simulink model "sm_vehicle_2axle_heave_roll_vtk"  (R2023b)
settings: Solver=ode1  StartTime=0.0  StopTime=inf  FixedStep=0.001  MaxStep=0.2  RelTol=1e-3  AbsTol=1e-3  EnableMultiTasking=on
PostLoadFcn:
  | if any(exist('dsrtsu_mdlpostloadfcn', 'file') ~= 0), dsrtsu_mdlpostloadfcn('Execute', bdroot); end
  | sm_vehicle_2axle_heave_roll_param
  | sm_vehicle_2axle_heave_roll_scene
  | sm_vehicle_2axle_heave_roll_config_maneuver(bdroot,VehicleData,'external');
InitFcn:
  | , if any(exist('rtifpga_mdlclblib', 'file') ~= 0), rtifpga_mdlclblib('Init', bdroot); end,
  | , if any(exist('dsmpb_private', 'file') ~= 0), dsmpb_private('dsmpb_mdlclblib', 'Init', bdroot); end,
StartFcn:
  | tic
StopFcn:
  | Elapsed_Sim_Time = toc;
undefined symbols (not defined in the file): InitVehicle, Maneuver, SceneData, trqFL, trqFR, trqRL, trqRR, VehicleData, VehicleData_P, X, Y, Z
libraries: sm_lib x62, nesl_utility x35, sm_vehicle_utilities_lib x18
(part 1 of 3)
PreSaveFcn:
  | , if any(exist('dsmpb_private', 'file') ~= 0), dsmpb_private('dsmpb_mdlclblib', 'PreSave', bdroot); end,
CloseFcn:
  | , if any(exist('dsmpb_private', 'file') ~= 0), dsmpb_private('dsmpb_mdlclblib', 'Close', bdroot); end,
  | try,close(h1_sm_vehicle_2axle_heave_roll),end
  | clear h1_sm_vehicle_2axle_heave_roll
  | try,close(h2_sm_vehicle_2axle_heave_roll),end
  | clear h2_sm_vehicle_2axle_heave_roll
  | try,close(h3_sm_vehicle_2axle_heave_roll),end
  | clear h3_sm_vehicle_2axle_heave_roll
  | 
  | 
  | clear simlog_sm_vehicle_2axle_heave_roll
  | clear logsout_sm_vehicle_2axle_heave_roll
Description:
  | Vehicle Dynamics, 14 DOF Model (Heave and Roll DOFs Per Axle)
  | 
  | Copyright 2022-2023 The MathWorks, Inc.
settings Model: DSMPB_ID_DATA={}  DSRTSU_INTERNAL_RTIFPGA=210  DSRTSU_INTERNAL_RTISTBM_VER=23.2  TunableVars=InitVehicle  TunableVarsStorageClass=ExportedGlobal  Creator=smiller  LastModifiedBy=matlabuser2
settings SolverCC: AutoScaleAbsTol=off  AlgebraicLoopSolver=TrustRegion
settings DataIOCC: SaveFormat=Array  SaveOutput=off  ReturnWorkspaceOutputs=off  SignalLoggingName=logsout_sm_vehicle_2axle_heave_roll_vtk  OutputTimes=[0:0.01:10]
settings OptimizationCC: DefaultParameterBehavior=Inlined  EnhancedBackFolding=on  ExpressionDepthLimit=2147483647  OptimizeBlockOrder=speed  DifferentSizesBufferReuse=on  OptimizationCustomize=off  EfficientTunableParamExpr=on
settings DebuggingCC: MergeDetectMultiDrivingBlocksExec=none  SolverPrmCheckMsg=warning  ParameterTunabilityLossMsg=error  UnconnectedInputMsg=warning  UnconnectedOutputMsg=warning  UnconnectedLineMsg=warning  StateNameClashWarn=warning  PregeneratedLibrarySubsystemCodeDiagnostic=none  SFUnexpectedBacktrackingDiag=warning  SFNoUnconditionalDefaultTransitionDiag=warning  SFExecutionAtInitializationDiag=none  ArithmeticOperatorsInVariantConditions=warning
settings HardwareCC: ProdBitPerPointer=32  ProdBitPerSizeT=32  ProdBitPerPtrDiffT=32  ProdLargestAtomicFloat=None  ProdIntDivRoundTo=Undefined  ProdEndianess=Unspecified  ProdWordSize=32  ProdHWDeviceType=32-bit Generic  TargetBitPerPointer=64  TargetBitPerSizeT=64  TargetBitPerPtrDiffT=64  TargetLongLongMode=on  TargetIntDivRoundTo=Zero  TargetEndianess=LittleEndian  TargetWordSize=64  TargetHWDeviceType=MATLAB Host  ProdEqTarget=off
settings ModelReferenceCC: EnableRefExpFcnMdlSchedulingChecks=on  PropagateSignalLabelsOutOfModel=off
settings SFSimCC: SimUseLocalCustomCode=off  MATLABDynamicMemAlloc=off  CustomCodeUndefinedFunction=UseInterfaceOnly
settings RTWCC: Description=Embedded Coder (host-based shared library target)  SystemTargetFile=ert_shrlib.tlc  TemplateMakefile=ert_default_tmf  RTWUseLocalCustomCode=off  BuildConfiguration=Faster Runs  DLArmComputeVersion=19.05
settings CodeAppCC: ForceParamTrailComments=on  IgnoreCustomStorageClasses=off  OperatorAnnotations=on  SimulinkDataObjDesc=on  SFDataObjDesc=on  InsertBlockDesc=on
settings STFCustomTargetCC: TargetLangStandard=C89/C90 (ANSI)  MultiwordLength=256  GenerateSampleERTMain=on  ParMdlRefBuildCompliant=on  CompOptLevelCompliant=on  CombineOutputUpdateFcns=on  ERTCustomFileBanners=on  CodeInterfacePackaging=Reusable function  SupportNonInlinedSFcns=off  RemoveResetFunc=on  MATLABClassNameForMDSCustomization=Simulink.SoftwareTarget.ERTCustomization  ModelStepFunctionPrototypeControlCompliant=on  UseToolchainInfoCompliant=on  SystemTargetFile=ert_shrlib.tlc
settings ERTTargetCC: GenerateSampleERTMain=on  ConcurrentExecutionCompliant=off  CodeInterfacePackaging=Reusable function  SupportContinuousTime=on  CPPClassGenCompliant=off  InlinedParameterPlacement=NonHierarchical  RootIOFormat=Structure reference  ERTCustomFileTemplate=example_file_process.tlc
settings ConfigComp: CovMetricSettings=dw  CovSaveCumulativeToWorkspaceVar=on  CovSaveSingleToWorkspaceVar=on  CovExternalEMLEnable=off
settings SimscapeCC: SimscapeNormalizeSystem=off  SimscapeLogType=all  SimscapeLogToSDI=on  SimscapeLogName=simlog_sm_vehicle_2axle_heave_roll
settings ConfigurationSet: Description=SimMechanics 2G
settings DiagnosticsConfigSet: SimMechanicsUnconnectedFramePorts=none  SimMechanicsConflictingReferenceFrames=none
settings ExplorerConfigSet: InternalSimMechanicsExplorerSettings="<ExplorerConfiguration><canonicalview>default</canonicalview><AnimationSetting><BasePlaybackSpeed>1.0</BasePlaybackSpeed><PlaybackSpeedFactor>2.0</PlaybackSpeedFactor></AnimationSetting><TilePanel><TileInfo><Tiles Columns=\"2\" Count=\"3\" Rows=\"2\"><Column Weight=\"0.6147\"/><Column Weight=\"0.3853\"/><Row Weight=\"0.3693\"/><Row Weight=\"0.6307\"/><Tile Height=\"1\" Width=\"1\" X=\"0\" Y=\"0\"/><Tile Height=\"1\" Width=\"1\" X=\"0\" Y=\"1\"/><Tile Height=\"2\" Width=\"1\" X=\"1\" Y=\"0\"/></Tiles></TileInfo><SceneInfo><SceneViewer><BGColor><R>1</R><G>1</G><B>1</B></BGColor><Camera><DoPerspective>on</DoPerspective><Position><X>-1.49999999999999911</X><Y>1.54074395550978868e-32</Y><Z>10.6999999999999993</Z></Position><Center><X>-1.49999999999999911</X><Y>1.54074395550978868e-32</Y><Z>9.69999999999999929</Z></Center><Up><X>0</X><Y>1</Y><Z>0</Z></Up><ViewLimDist>1</ViewLimDist><YLim>0.466307658154998583</YLim><XLim>1.34838716914770518</XLim></Camera></SceneViewer><SceneViewer><BGColor><R>1</R><G>1</G><B>1</B></BGColor><Camera><DoPerspective>on</DoPerspective><Position><X>2.34000000000000163</X><Y>-3.20000000000000151</Y><Z>1.80000000000000004</Z></Position><Center><X>1.58973091910295716</X><Y>-2.57477576591913149</Y><Z>1.58507916953470085</Z></Center><Up><X>-0.16510675539218278</X><Y>0.137588962826818928</Y><Z>0.976631474319820447</Z></Up><ViewLimDist>1</ViewLimDist><YLim>0.466307658154998583</YLim><XLim>0.779836453951521791</XLim></Camera></SceneViewer><SceneViewer><BGColor><R>1</R><G>1</G><B>1</B></BGColor><Camera><DoPerspective>on</DoPerspective><Position><X>-6.5</X><Y>3.46944695195361419e-16</Y><Z>1.79999999999999982</Z></Position><Center><X>-5.52335553329491002</X><Y>3.46944695195361419e-16</Y><Z>1.58513821732488003</Z></Center><Up><X>0.214861782675119795</X><Y>-1.71056941445900502e-49</Y><Z>0.976644466705089975</Z></Up><ViewLimDist>1</ViewLimDist><YLim>0.466307658154998583</YLim><XLim>0.303969645724483983</XLim></Camera></SceneViewer></SceneInfo></TilePanel><MechEditorPanel><Cameras><Camera><Id>Camera1</Id><Value><Name>Track FixO FR</Name><NativeCamera><PositionTrackingFeature>Vehicle.Camera_Frames.Frame_FixO_FR.R</PositionTrackingFeature><CenterTrackingFeature>Vehicle.Camera_Frames.Frame_FixO_FR.R</CenterTrackingFeature><UpVectorTrackingFeature>Vehicle.Camera_Frames.Frame_FixO_FR.R</UpVectorTrackingFeature><CenterTrackingOrigin>off</CenterTrackingOrigin><CenterTrackingDirection>+X</CenterTrackingDirection><UpVectorTrackingDirection>+Z</UpVectorTrackingDirection></NativeCamera></Value></Camera><Camera><Id>Camera2</Id><Value><Name>Track FixO Right</Name><NativeCamera><PositionTrackingFeature>Vehicle.Camera_Frames.Frame_FixO_Right.R</PositionTrackingFeature><CenterTrackingFeature>Vehicle.Camera_Frames.Frame_FixO_Right.R</CenterTrackingFeature><UpVectorTrackingFeature>Vehicle.Camera_Frames.Frame_FixO_Right.R</UpVectorTrackingFeature><CenterTrackingOrigin>off</CenterTrackingOrigin><CenterTrackingDirection>+X</CenterTrackingDirection><UpVectorTrackingDirection>+Z</UpVectorTrackingDirection></NativeCamera></Value></Camera><Camera><Id>Camera3</Id><Value><Name>Track FixO RR</Name><NativeCamera><PositionTrackingFeature>Vehicle.Camera_Frames.Frame_FixO_RR.R</PositionTrackingFeature><CenterTrackingFeature>Vehicle.Camera_Frames.Frame_FixO_RR.R</CenterTrackingFeature><UpVectorTrackingFeature>Vehicle.Camera_Frames.Frame_FixO_RR.R</UpVectorTrackingFeature><CenterTrackingOrigin>off</CenterTrackingOrigin><CenterTrackingDirection>+X</CenterTrackingDirection><UpVectorTrackingDirection>+Z</UpVectorTrackingDirection></NativeCamera></Value></Camera><Camera><Id>Camera4</Id><Value><Name>Track FixO RL</Name><NativeCamera><PositionTrackingFeature>Vehicle.Camera_Frames.Frame_FixO_RL.R</PositionTrackingFeature><CenterTrackingFeature>Vehicle.Camera_Frames.Frame_FixO_RL.R</CenterTrackingFeature><UpVectorTrackingFeature>Vehicle.Camera_Frames.Frame_FixO_RL.R</UpVectorTrackingFeature><CenterTrackingOrigin>off</CenterTrackingOrigin><CenterTrackingDirection>+X</CenterTrackingDirection><UpVectorTrackingDirection>+Z</UpVectorTrackingDirection></NativeCamera></Value></Camera><Camera><Id>Camera5</Id><Value><Name>Track FixO Left</Name><NativeCamera><PositionTrackingFeature>Vehicle.Camera_Frames.Frame_FixO_Left.R</PositionTrackingFeature><CenterTrackingFeature>Vehicle.Camera_Frames.Frame_FixO_Left.R</CenterTrackingFeature><UpVectorTrackingFeature>Vehicle.Camera_Frames.Frame_FixO_Left.R</UpVectorTrackingFeature><CenterTrackingOrigin>off</CenterTrackingOrigin><CenterTrackingDirection>+X</CenterTrackingDirection><UpVectorTrackingDirection>+Z</UpVectorTrackingDirection></NativeCamera></Value></Camera><Camera><Id>Camera6</Id><Value><Name>Track FixO FL</Name><NativeCamera><PositionTrackingFeature>Vehicle.Camera_Frames.Frame_FixO_FL.R</PositionTrackingFeature><CenterTrackingFeature>Vehicle.Camera_Frames.Frame_FixO_FL.R</CenterTrackingFeature><UpVectorTrackingFeature>Vehicle.Camera_Frames.Frame_FixO_FL.R</UpVectorTrackingFeature><CenterTrackingOrigin>off</CenterTrackingOrigin><CenterTrackingDirection>+X</CenterTrackingDirection><UpVectorTrackingDirection>+Z</UpVectorTrackingDirection></NativeCamera></Value></Camera><Camera><Id>Camera7</Id><Value><Name>Track FixO Top</Name><NativeCamera><PositionTrackingFeature>Vehicle.Camera_Frames.Frame_FixO_Top.R</PositionTrackingFeature><CenterTrackingFeature>Vehicle.Camera_Frames.Frame_FixO_Top.R</CenterTrackingFeature><UpVectorTrackingFeature>Vehicle.Camera_Frames.Frame_FixO_Top.R</UpVectorTrackingFeature><CenterTrackingOrigin>off</CenterTrackingOrigin><CenterTrackingDirection>+X</CenterTrackingDirection><UpVectorTrackingDirection>+Z</UpVectorTrackingDirection></NativeCamera></Value></Camera><Camera><Id>Camera8</Id><Value><Name>Track FixO Front</Name><NativeCamera><PositionTrackingFeature>Vehicle.Camera_Frames.Frame_FixO_Front.R</PositionTrackingFeature><CenterTrackingFeature>Vehicle.Camera_Frames.Frame_FixO_Front.R</CenterTrackingFeature><UpVectorTrackingFeature>Vehicle.Camera_Frames.Frame_FixO_Front.R</UpVectorTrackingFeature><CenterTrackingOrigin>off</CenterTrackingOrigin><CenterTrackingDirection>+X</CenterTrackingDirection><UpVectorTrackingDirection>+Z</UpVectorTrackingDirection></NativeCamera></Value></Camera><Camera><Id>Camera9</Id><Value><Name>Track FixO Rear</Name><NativeCamera><PositionTrackingFeature>Vehicle.Camera_Frames.Frame_FixO_Rear.R</PositionTrackingFeature><CenterTrackingFeature>Vehicle.Camera_Frames.Frame_FixO_Rear.R</CenterTrackingFeature><UpVectorTrackingFeature>Vehicle.Camera_Frames.Frame_FixO_Rear.R</UpVectorTrackingFeature><CenterTrackingOrigin>off</CenterTrackingOrigin><CenterTrackingDirection>+X</CenterTrackingDirection><UpVectorTrackingDirection>+Z</UpVectorTrackingDirection></NativeCamera></Value></Camera><Camera><Id>Camera10</Id><Value><Name>Track FR</Name><NativeCamera><PositionTrackingFeature>Vehicle.Camera_Frames.Frame_FR.R</PositionTrackingFeature><CenterTrackingFeature>Vehicle.Camera_Frames.Frame_FR.R</CenterTrackingFeature><UpVectorTrackingFeature>Vehicle.Camera_Frames.Frame_FR.R</UpVectorTrackingFeature><CenterTrackingOrigin>off</CenterTrackingOrigin><CenterTrackingDirection>+X</CenterTrackingDirection><UpVectorTrackingDirection>+Z</UpVectorTrackingDirection></NativeCamera></Value></Camera><Camera><Id>Camera11</Id><Value><Name>Track Right</Name><NativeCamera><PositionTrackingFeature>Vehicle.Camera_Frames.Frame_Right.R</PositionTrackingFeature><CenterTrackingFeature>Vehicle.Camera_Frames.Frame_Right.R</CenterTrackingFeature><UpVectorTrackingFeature>Vehicle.Camera_Frames.Frame_Right.R</UpVectorTrackingFeature><CenterTrackingOrigin>off</CenterTrackingOrigin><CenterTrackingDirection>+X</CenterTrackingDirection><UpVectorTrackingDirection>+Z</UpVectorTrackingDirection></NativeCamera></Value></Camera><Camera><Id>Camera12</Id><Value><Name>Track RR</Name><NativeCamera><PositionTrackingFeature>Vehicle.Camera_Frames.Frame_RR.R</PositionTrackingFeature><CenterTrackingFeature>Vehicle.Camera_Frames.Frame_RR.R</CenterTrackingFeature><UpVectorTrackingFeature>Vehicle.Camera_Frames.Frame_RR.R</UpVectorTrackingFeature><CenterTrackingOrigin>off</CenterTrackingOrigin><CenterTrackingDirection>+X</CenterTrackingDirection><UpVectorTrackingDirection>+Z</UpVectorTrackingDirection></NativeCamera></Value></Camera><Camera><Id>Camera13</Id><Value><Name>Track RL</Name><NativeCamera><PositionTrackingFeature>Vehicle.Camera_Frames.Frame_RL.R</PositionTrackingFeature><CenterTrackingFeature>Vehicle.Camera_Frames.Frame_RL.R</CenterTrackingFeature><UpVectorTrackingFeature>Vehicle.Camera_Frames.Frame_RL.R</UpVectorTrackingFeature><CenterTrackingOrigin>off</CenterTrackingOrigin><CenterTrackingDirection>+X</CenterTrackingDirection><UpVectorTrackingDirection>+Z</UpVectorTrackingDirection></NativeCamera></Value></Camera><Camera><Id>Camera14</Id><Value><Name>Track Left</Name><NativeCamera><PositionTrackingFeature>Vehicle.Camera_Frames.Frame_Left.R</PositionTrackingFeature><CenterTrackingFeature>Vehicle.Camera_Frames.Frame_Left.R</CenterTrackingFeature><UpVectorTrackingFeature>Vehicle.Camera_Frames.Frame_Left.R</UpVectorTrackingFeature><CenterTrackingOrigin>off</CenterTrackingOrigin><CenterTrackingDirection>+X</CenterTrackingDirection><UpVectorTrackingDirection>+Z</UpVectorTrackingDirection></NativeCamera></Value></Camera><Camera><Id>Camera15</Id><Value><Name>Track FL</Name><NativeCamera><PositionTrackingFeature>Vehicle.Camera_Frames.Frame_FL.R</PositionTrackingFeature><CenterTrackingFeature>Vehicle.Camera_Frames.Frame_FL.R</CenterTrackingFeature><UpVectorTrackingFeature>Vehicle.Camera_Frames.Frame_FL.R</UpVectorTrackingFeature><CenterTrackingOrigin>off</CenterTrackingOrigin><CenterTrackingDirection>+X</CenterTrackingDirection><UpVectorTrackingDirection>+Z</UpVectorTrackingDirection></NativeCamera></Value></Camera><Camera><Id>Camera16</Id><Value><Name>Track Top</Name><NativeCamera><PositionTrackingFeature>Vehicle.Camera_Frames.Frame_Top.R</PositionTrackingFeature><CenterTrackingFeature>Vehicle.Camera_Frames.Frame_Top.R</CenterTrackingFeature><UpVectorTrackingFeature>Vehicle.Camera_Frames.Frame_Top.R</UpVectorTrackingFeature><CenterTrackingOrigin>off</CenterTrackingOrigin><CenterTrackingDirection>+X</CenterTrackingDirection><UpVectorTrackingDirection>+Z</UpVectorTrackingDirection></NativeCamera></Value></Camera><Camera><Id>Camera17</Id><Value><Name>Track Front</Name><NativeCamera><PositionTrackingFeature>Vehicle.Camera_Frames.Frame_Front.R</PositionTrackingFeature><CenterTrackingFeature>Vehicle.Camera_Frames.Frame_Front.R</CenterTrackingFeature><UpVectorTrackingFeature>Vehicle.Camera_Frames.Frame_Front.R</UpVectorTrackingFeature><CenterTrackingOrigin>off</CenterTrackingOrigin><CenterTrackingDirection>+X</CenterTrackingDirection><UpVectorTrackingDirection>+Z</UpVectorTrackingDirection></NativeCamera></Value></Camera><Camera><Id>Camera18</Id><Value><Name>Track Rear</Name><NativeCamera><PositionTrackingFeature>Vehicle.Camera_Frames.Frame_Rear.R</PositionTrackingFeature><CenterTrackingFeature>Vehicle.Camera_Frames.Frame_Rear.R</CenterTrackingFeature><UpVectorTrackingFeature>Vehicle.Camera_Frames.Frame_Rear.R</UpVectorTrackingFeature><CenterTrackingOrigin>off</CenterTrackingOrigin><CenterTrackingDirection>+X</CenterTrackingDirection><UpVectorTrackingDirection>+Z</UpVectorTrackingDirection></NativeCamera></Value></Camera><Camera><Id>Camera19</Id><Value><Name>Track SuspF</Name><NativeCamera><PositionTrackingFeature>Vehicle.Camera_Frames.Frame_SuspF.R</PositionTrackingFeature><CenterTrackingFeature>Vehicle.Camera_Frames.Frame_SuspF.R</CenterTrackingFeature><UpVectorTrackingFeature>Vehicle.Camera_Frames.Frame_SuspF.R</UpVectorTrackingFeature><CenterTrackingOrigin>off</CenterTrackingOrigin><CenterTrackingDirection>+X</CenterTrackingDirection><UpVectorTrackingDirection>+Z</UpVectorTrackingDirection></NativeCamera></Value></Camera><Camera><Id>Camera20</Id><Value><Name>Track SuspR</Name><NativeCamera><PositionTrackingFeature>Vehicle.Camera_Frames.Frame_SuspR.R</PositionTrackingFeature><CenterTrackingFeature>Vehicle.Camera_Frames.Frame_SuspR.R</CenterTrackingFeature><UpVectorTrackingFeature>Vehicle.Camera_Frames.Frame_SuspR.R</UpVectorTrackingFeature><CenterTrackingOrigin>off</CenterTrackingOrigin><CenterTrackingDirection>+X</CenterTrackingDirection><UpVectorTrackingDirection>+Z</UpVectorTrackingDirection></NativeCamera></Value></Camera><Camera><Id>Camera21</Id><Value><Name>Track WheelFR</Name><NativeCamera><PositionTrackingFeature>Vehicle.Camera_Frames.Frame_Wheel_FR.R</PositionTrackingFeature><CenterTrackingFeature>Vehicle.Camera_Frames.Frame_Wheel_FR.R</CenterTrackingFeature><UpVectorTrackingFeature>Vehicle.Camera_Frames.Frame_Wheel_FR.R</UpVectorTrackingFeature><CenterTrackingOrigin>off</CenterTrackingOrigin><CenterTrackingDirection>+X</CenterTrackingDirection><UpVectorTrackingDirection>+Z</UpVectorTrackingDirection></NativeCamera></Value></Camera><Camera><Id>Camera22</Id><Value><Name>Track WheelRR</Name><NativeCamera><PositionTrackingFeature>Vehicle.Camera_Frames.Frame_Wheel_RR.R</PositionTrackingFeature><CenterTrackingFeature>Vehicle.Camera_Frames.Frame_Wheel_RR.R</CenterTrackingFeature><UpVectorTrackingFeature>Vehicle.Camera_Frames.Frame_Wheel_RR.R</UpVectorTrackingFeature><CenterTrackingOrigin>off</CenterTrackingOrigin><CenterTrackingDirection>+X</CenterTrackingDirection><UpVectorTrackingDirection>+Z</UpVectorTrackingDirection></NativeCamera></Value></Camera><Camera><Id>Camera23</Id><Value><Name>Track WheelRL</Name><NativeCamera><PositionTrackingFeature>Vehicle.Camera_Frames.Frame_Wheel_RL.R</PositionTrackingFeature><CenterTrackingFeature>Vehicle.Camera_Frames.Frame_Wheel_RL.R</CenterTrackingFeature><UpVectorTrackingFeature>Vehicle.Camera_Frames.Frame_Wheel_RL.R</UpVectorTrackingFeature><CenterTrackingOrigin>off</CenterTrackingOrigin><CenterTrackingDirection>+X</CenterTrackingDirection><UpVectorTrackingDirection>+Z</UpVectorTrackingDirection></NativeCamera></Value></Camera><Camera><Id>Camera24</Id><Value><Name>Track WheelFL</Name><NativeCamera><PositionTrackingFeature>Vehicle.Camera_Frames.Frame_Wheel_FL.R</PositionTrackingFeature><CenterTrackingFeature>Vehicle.Camera_Frames.Frame_Wheel_FL.R</CenterTrackingFeature><UpVectorTrackingFeature>Vehicle.Camera_Frames.Frame_Wheel_FL.R</UpVectorTrackingFeature><CenterTrackingOrigin>off</CenterTrackingOrigin><CenterTrackingDirection>+X</CenterTrackingDirection><UpVectorTrackingDirection>+Z</UpVectorTrackingDirection></NativeCamera></Value></Camera><Camera><Id>Camera25</Id><Value><Name>View Seat FL</Name><NativeCamera><PositionTrackingFeature>Vehicle.Camera_Frames.Frame_View_Seat_FL.R</PositionTrackingFeature><CenterTrackingFeature>Vehicle.Camera_Frames.Frame_View_Seat_FL.R</CenterTrackingFeature><UpVectorTrackingFeature>Vehicle.Camera_Frames.Frame_View_Seat_FL.R</UpVectorTrackingFeature><CenterTrackingOrigin>off</CenterTrackingOrigin><CenterTrackingDirection>+X</CenterTrackingDirection><UpVectorTrackingDirection>+Z</UpVectorTrackingDirection></NativeCamera></Value></Camera><Camera><Id>Camera26</Id><Value><Name>View Seat FR</Name><NativeCamera><PositionTrackingFeature>Vehicle.Camera_Frames.Frame_View_Seat_FR.R</PositionTrackingFeature><CenterTrackingFeature>Vehicle.Camera_Frames.Frame_View_Seat_FR.R</CenterTrackingFeature><UpVectorTrackingFeature>Vehicle.Camera_Frames.Frame_View_Seat_FR.R</UpVectorTrackingFeature><CenterTrackingOrigin>off</CenterTrackingOrigin><CenterTrackingDirection>+X</CenterTrackingDirection><UpVectorTrackingDirection>+Z</UpVectorTrackingDirection></NativeCamera></Value></Camera><Camera><Id>Camera27</Id><Value><Name>View Susp FR</Name><NativeCamera><PositionTrackingFeature>Vehicle.Camera_Frames.Frame_View_Susp_FR.R</PositionTrackingFeature><CenterTrackingFeature>Vehicle.Camera_Frames.Frame_View_Susp_FR.R</CenterTrackingFeature><UpVectorTrackingFeature>Vehicle.Camera_Frames.Frame_View_Susp_FR.R</UpVectorTrackingFeature><CenterTrackingOrigin>off</CenterTrackingOrigin><CenterTrackingDirection>+X</CenterTrackingDirection><UpVectorTrackingDirection>+Z</UpVectorTrackingDirection></NativeCamera></Value></Camera><Camera><Id>Camera28</Id><Value><Name>View Susp RR</Name><NativeCamera><PositionTrackingFeature>Vehicle.Camera_Frames.Frame_View_Susp_RR.R</PositionTrackingFeature><CenterTrackingFeature>Vehicle.Camera_Frames.Frame_View_Susp_RR.R</CenterTrackingFeature><UpVectorTrackingFeature>Vehicle.Camera_Frames.Frame_View_Susp_RR.R</UpVectorTrackingFeature><CenterTrackingOrigin>off</CenterTrackingOrigin><CenterTrackingDirection>+X</CenterTrackingDirection><UpVectorTrackingDirection>+Z</UpVectorTrackingDirection></NativeCamera></Value></Camera><Camera><Id>Camera29</Id><Value><Name>View Susp RL</Name><NativeCamera><PositionTrackingFeature>Vehicle.Camera_Frames.Frame_View_Susp_RL.R</PositionTrackingFeature><CenterTrackingFeature>Vehicle.Camera_Frames.Frame_View_Susp_RL.R</CenterTrackingFeature><UpVectorTrackingFeature>Vehicle.Camera_Frames.Frame_View_Susp_RL.R</UpVectorTrackingFeature><CenterTrackingOrigin>off</CenterTrackingOrigin><CenterTrackingDirection>+X</CenterTrackingDirection><UpVectorTrackingDirection>+Z</UpVectorTrackingDirection></NativeCamera></Value></Camera><Camera><Id>Camera30</Id><Value><Name>View Susp FL</Name><NativeCamera><PositionTrackingFeature>Vehicle.Camera_Frames.Frame_View_Susp_FL.R</PositionTrackingFeature><CenterTrackingFeature>Vehicle.Camera_Frames.Frame_View_Susp_FL.R</CenterTrackingFeature><UpVectorTrackingFeature>Vehicle.Camera_Frames.Frame_View_Susp_FL.R</UpVectorTrackingFeature><CenterTrackingOrigin>off</CenterTrackingOrigin><CenterTrackingDirection>+X</CenterTrackingDirection><UpVectorTrackingDirection>+Z</UpVectorTrackingDirection></NativeCamera></Value></Camera><Camera><Id>Camera31</Id><Value><Name>Dolly Camera</Name><NativeCamera><PositionTrackingFeature>Vehicle.Camera_Frames.Frame_Dolly.R</PositionTrackingFeature><CenterTrackingFeature>Vehicle.Camera_Frames.Frame_Dolly.R</CenterTrackingFeature><UpVectorTrackingFeature>Vehicle.Camera_Frames.Frame_Dolly.R</UpVectorTrackingFeature><CenterTrackingOrigin>off</CenterTrackingOrigin><CenterTrackingDirection>+X</CenterTrackingDirection><UpVectorTrackingDirection>+Z</UpVectorTrackingDirection></NativeCamera></Value></Camera><Camera><Id>Camera32</Id><Value><Name>Track Dolly Camera</Name><NativeCamera><PositionTrackingFeature>Vehicle.Camera_Frames.Frame_Dolly.R</PositionTrackingFeature><CenterTrackingFeature>Vehicle.Camera_Frames.Transform_Camera_Ref.F</CenterTrackingFeature><UpVectorTrackingFeature>Vehicle.Camera_Frames.World_Frame.W</UpVectorTrackingFeature><CenterTrackingOrigin>on</CenterTrackingOrigin><UpVectorTrackingDirection>+Z</UpVectorTrackingDirection></NativeCamera></Value></Camera></Cameras><GfxPanelCameraMap><MapElement CameraMLId=\"Camera7\" GfxPanelIndex=\"0\"/><MapElement CameraMLId=\"Camera1\" GfxPanelIndex=\"1\"/><MapElement CameraMLId=\"Camera9\" GfxPanelIndex=\"2\"/></GfxPanelCameraMap><VideoCreator><PlaybackSpeedRatio>1.0</PlaybackSpeedRatio><FrameRate>30</FrameRate><VideoFormat>MPEG-4</VideoFormat><FrameSize>[800 450]</FrameSize></VideoCreator></MechEditorPanel></ExplorerConfiguration>"

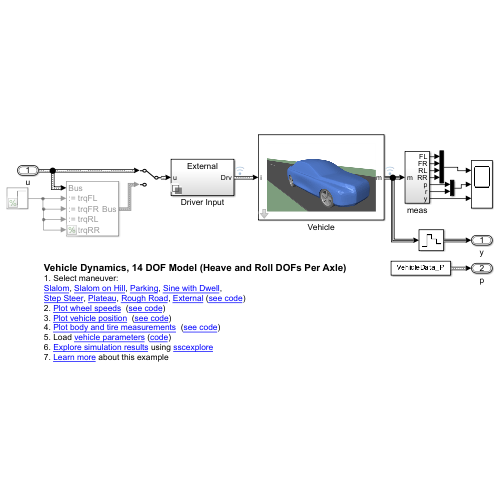
[thumbnail: Simulink's stored preview of the top-level diagram]
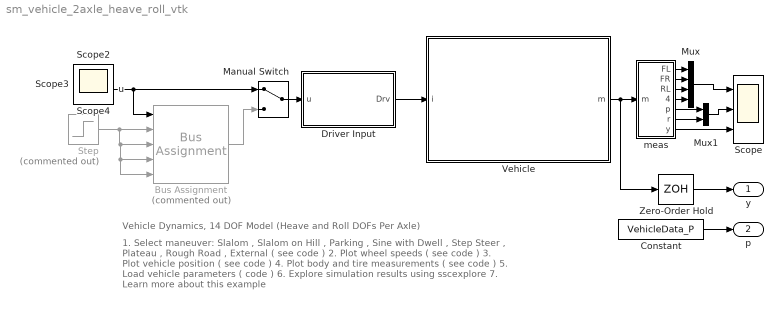
== system sm_vehicle_2axle_heave_roll_vtk ==
  note: Vehicle Dynamics, 14 DOF Model (Heave and Roll DOFs Per Axle)
  note: 1. Select maneuver:
      | Slalom , Slalom on Hill , Parking , Sine with Dwell ,
      | Step Steer , Plateau , Rough Road , External ( see code )
      | 2. Plot wheel speeds ( see code )
      | 3. Plot vehicle position ( see code )
      | 4. Plot body and tire measurements ( see code )
      | 5. Load vehicle parameters ( code )
      | 6. Explore simulation results using sscexplore
      | 7. Learn more about this example
  u : Inport  OutDataTypeStr=Bus: sm_vehicle_2axle_heave_roll_U_t  BusOutputAsStruct=on
  Bus Assignment : BusAssignment  Commented=on  AssignedSignals=trqFL,trqFR,trqRL,trqRR
  Constant : Constant  Value=VehicleData_P  VectorParams1D=off  OutDataTypeStr=Bus: VehicleData_t
  Driver Input : Subsystem  Variant=on  VariantControlMode=label  LabelModeActiveChoice=External
  Manual Switch : ManualSwitch
  Mux : Mux
  Mux1 : Mux  Inputs=2
  Scope : Scope  NumInputPorts=3
  Step : Step  Commented=on  After=1000  SampleTime=0
  Vehicle : Subsystem  mask(Vehicle and Scene){vehdata=VehicleData, initveh=InitVehicle, popup_scene=Grid, popup_road_surface=Flat}
      mask prompts: vehdata "Vehicle Data (structure)"; initveh "Initial Position, Velocity (structure)"; popup_scene "Scene"; popup_road_surface "Road Surface"
      mask help: Models a vehicle with a configurable scene. Vehicle parameters are defined within a single data structure. A separate data structure defines the initial position, orientation, and speed of the vehicle and the wheels.
      mask init:
      | scene_name = strrep(get_param(gcb,'popup_scene'),' ','_');
      | set_param([gcb '/Scene'],'LabelModeActiveChoice',scene_name);
      | surface_name = strrep(get_param(gcb,'popup_road_surface'),' ','_');
      | set_param([gcb '/Road Surface FL'],'LabelModeActiveChoice',surface_name);
      | set_param([gcb '/Road Surface FR'],'LabelModeActiveChoice',surface_name);
      | set_param([gcb '/Road Surface RL'],'LabelModeActiveChoice',surface_name);
      | set_param([gcb '/Road Surface RR'],'LabelModeActiveChoice',surface_name);
      mask TypeOptions popup_scene: Grid | Road | Plateau | Rough Road | None
      mask TypeOptions popup_road_surface: Flat | Plateau | Rough Road
      mask Display: image('sm_vehicle_2axle_heave_roll_vehicle_scene.png');
  Zero-Order Hold : ZeroOrderHold  SampleTime=-1
  meas : Subsystem
  y : Outport  OutDataTypeStr=Bus: sm_vehicle_2axle_heave_roll_Y_t  BusOutputAsStruct=on
  p : Outport  Port=2  OutDataTypeStr=Bus: VehicleData_t  BusOutputAsStruct=on
  Scope2 : Scope
  Scope3 : Scope
  Scope4 : Scope
  wires:
  Driver Input/1(Drv) -> Vehicle/1(i)
  Vehicle/1(m) -> Zero-Order Hold/1, meas/1(m)
  Mux/1 -> Scope/1
  meas/1(FL) -> Mux/1
  meas/2(FR) -> Mux/2
  meas/3(RL) -> Mux/3
  meas/4(RR) -> Mux/4
  meas/5(p) -> Mux1/1
  meas/6(r) -> Mux1/2
  Mux1/1 -> Scope/2
  meas/7(y) -> Scope/3
  u/1 -> Bus Assignment/1, Manual Switch/1
  Manual Switch/1 -> Driver Input/1(u)
  Bus Assignment/1 -> Manual Switch/2
  Step/1 -> Bus Assignment/5, Bus Assignment/4, Bus Assignment/3, Bus Assignment/2
  Constant/1 -> p/1
  Zero-Order Hold/1 -> y/1

== system sm_vehicle_2axle_heave_roll_vtk/Driver Input ==
  u : Inport
  External : Subsystem  VariantControl=External
  No Steer : Subsystem  VariantControl=NoSteer
  Parking : Subsystem  VariantControl=Parking
  Sine With Dwell : Subsystem  VariantControl=SineWithDwell
  Slalom : Subsystem  VariantControl=Slalom
  Step Steer : Subsystem  VariantControl=StepSteer
  Drv : Outport

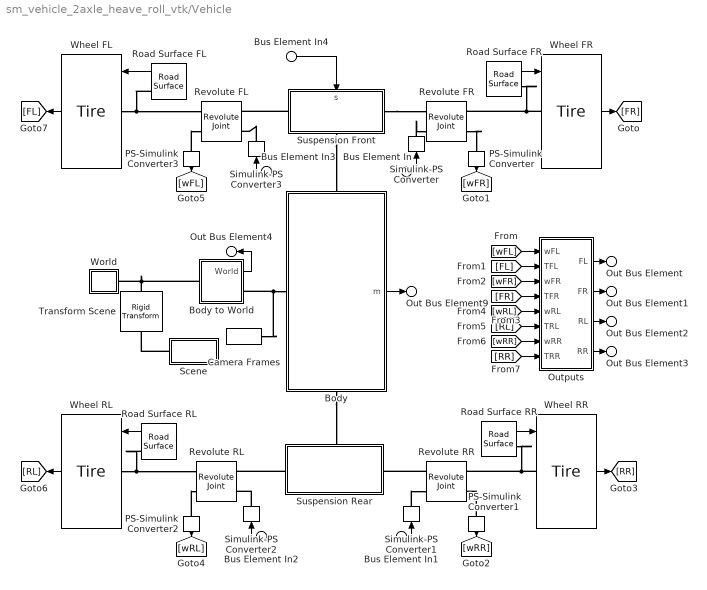
== system sm_vehicle_2axle_heave_roll_vtk/Vehicle ==
  Bus Element In : Inport  PortName=i  Element=trqFR
  Bus Element In1 : Inport  PortName=i  Element=trqRR
  Bus Element In2 : Inport  PortName=i  Element=trqRL
  Bus Element In3 : Inport  PortName=i  Element=trqFL
  Bus Element In4 : Inport  PortName=i  Element=sWhl
  Body : Subsystem  mask(Body for 2-Axle Vehicle){xRefToFA=vehdata.Body.FA, xRefToRA=vehdata.Body.RA, xyzRefToCG=vehdata.Body.CG, xyzRefToGeometry=vehdata.Body.Geometry, mBody=vehdata.Body.Mass, JBody=vehdata.Body.Inertias, clrBody=vehdata.Body.Color, opcBody=vehdata.Body.Opacity}
      mask prompts: xRefToFA "Offset Reference to Front Axle (m)"; xRefToRA "Offset Reference to Rear Axle (m)"; xyzRefToCG "Offset Reference to CG [x y z] (m)"; xyzRefToGeometry "Offset Reference to Geometry [x y z] (m)"; mBody "Body Mass (kg)"; JBody "Body Inertia [Ixx Iyy Izz] (kg*m^2)"; clrBody "Body Color [R G B]"; opcBody "Body Opacity (0-1)"
      mask help: Models mass and inertia of rigid vehicle body. Frames for front suspension, rear suspension, center of gravity, and body geometry are all defined relative to the reference frame. Measurements are with respect to the body frame.
      settings: PortSchema="{\"entries\":[{\"content\":{\"sides\":[{\"content\":{\"connectorIds\":[\"LConn1\"]},\"type\":\"ConnectorPlacement.EquallySpacedRectSide\",\"uuid\":\"a6a40084-0b01-416d-a19a-d775fde84bbf\"},{\"content\":{\"connectorIds\":[\"RConn1\"],\"side\":\"RIGHT\"},\"type\":\"ConnectorPlacement.EquallySpacedRectSide\",\"uuid\":\"7b527776-1265-46e3-b587-d37cab880183\"},{\"content\":{\"connectorIds\":[\"Out1\"],\"side\":\"TOP\"},\"type\":\"ConnectorPlacement.EquallySpacedRectSide\",\"uuid\":\"f01e2205-af4e-42ab-b4af-31b005ea0e61\"},{\"content\":{\"connectorIds\":[\"RConn2\"],\"side\":\"BOTTOM\"},\"type\":\"ConnectorPlacement.EquallySpacedRectSide\",\"uuid\":\"682a6e2c-9f3d-4bbb-bb88-e5eb72c2e6bf\"}]},\"type\":\"ConnectorPlacement.EquallySpacedConnector\",\"uuid\":\"a1282978-4c55-459b-9a00-856109b4503f\"}],\"packageUris\":[\"http://schema.mathworks.com/mf0/Connector/R2020b\"],\"version\":\"1.0\"}"
      mask Display: image('sm_vehicle_utilities_body_sedan.png');
  Body to World : Subsystem  AncestorBlock=sm_vehicle_utilities_lib/Body to World  mask(Body to World){Init=initveh.Vehicle, SpecifyPosTarget=on}
      mask prompts: Init "Initial Values"; SpecifyPosTarget "Specify Position Target"
      mask help: Models the connection between the vehicle body and world. Permits 6 degrees of freedom and sets the initial position, orientation, and speed of the vehicle body.
      mask init:
      | initial_aveh = [Init.yaw Init.pitch Init.roll];
      | rotmat_ypr = sm_vehicle_yawpitchroll_to_rotmat(Init.yaw, Init.pitch, Init.roll);
      | initial_vveh = rotmat_ypr*([Init.vx Init.vy Init.vz])';
      | 
      | sptState = get_param(gcb,'SpecifyPosTarget');
      | 
      | set_param([gcb '/Body World Joint'],...
      |         'PxPositionTargetSpecify',sptState,...
      |         'PyPositionTargetSpecify',sptState,...
      |         'PzPositionTargetSpecify',sptState,...
      |         'SphPositionTargetSpecify',sptState,...
      |         'PxVelocityTargetSpecify',sptState,...
      |         'PyVelocityTargetSpecify',sptState,...
      |         'PzVelocityTargetSpecify',sptState...
      |         );
      mask Help: web('sm_car_doc_body_to_world.html')
  Camera Frames : sm_vehicle_utilities_lib/Camera Frames  Camera=Camera  popup_dolly_camera=Off
  Outputs : Subsystem
  PS-Simulink Converter{,1..3} (4 alike) : nesl_utility/PS-Simulink Converter  PhysicalDomain=network_engine_domain  SubClassName=ps_output  LeftPortType=input  RightPortType=output  PseudoPeriodic=off  Frequencies=[]  VectorFormat=1-D array  Unit=inherit  AffineConversion=off
  Revolute FL : sm_lib/Joints/Revolute Joint  JointMode=Normal  SenseConstraintForce=off  SenseConstraintForceX=off  SenseConstraintForceY=off  SenseConstraintForceZ=off  SenseConstraintTorque=off  SenseConstraintTorqueX=off  SenseConstraintTorqueY=off  SenseConstraintTorqueZ=off  SenseTotalForce=off  SenseTotalForceX=off  SenseTotalForceY=off  SenseTotalForceZ=off  SenseTotalTorque=off  SenseTotalTorqueX=off  SenseTotalTorqueY=off  SenseTotalTorqueZ=off  CompositeWrenchDir=FollowerOnBase  CompositeWrenchFrame=BaseFrame  EquilibriumPosition=0  EquilibriumPositionUnits=rad  SpringStiffness=0  SpringStiffnessUnits=N*m/rad  DampingCoefficient=0  DampingCoefficientUnits=N*m/(rad/s)  TorqueActuationMode=InputTorque  MotionActuationMode=ComputedMotion  SensePosition=off  SenseVelocity=on  SenseAcceleration=off  SenseTorqueForce=off  SenseLowerLimitTorqueForce=off  SenseUpperLimitTorqueForce=off  LowerLimitSpecify=off  LowerLimitBound=-90  LowerLimitBoundUnits=deg  LowerLimitStiffness=1e4  LowerLimitStiffnessUnits=N*m/deg  LowerLimitDamping=10  LowerLimitDampingUnits=N*m/(deg/s)  LowerLimitTransitionRegionWidth=0.1  LowerLimitTransitionRegionWidthUnits=deg  UpperLimitSpecify=off  UpperLimitBound=90  UpperLimitBoundUnits=deg  UpperLimitStiffness=1e4  UpperLimitStiffnessUnits=N*m/deg  UpperLimitDamping=10  UpperLimitDampingUnits=N*m/(deg/s)  UpperLimitTransitionRegionWidth=0.1  UpperLimitTransitionRegionWidthUnits=deg  PositionTargetSpecify=off  PositionTargetPriority=High  PositionTargetValue=0  PositionTargetValueUnits=deg  VelocityTargetSpecify=on  VelocityTargetPriority=High  VelocityTargetValue=initveh.Wheel.wFL  VelocityTargetValueUnits=rad/s
  Revolute FR : sm_lib/Joints/Revolute Joint  JointMode=Normal  SenseConstraintForce=off  SenseConstraintForceX=off  SenseConstraintForceY=off  SenseConstraintForceZ=off  SenseConstraintTorque=off  SenseConstraintTorqueX=off  SenseConstraintTorqueY=off  SenseConstraintTorqueZ=off  SenseTotalForce=off  SenseTotalForceX=off  SenseTotalForceY=off  SenseTotalForceZ=off  SenseTotalTorque=off  SenseTotalTorqueX=off  SenseTotalTorqueY=off  SenseTotalTorqueZ=off  CompositeWrenchDir=FollowerOnBase  CompositeWrenchFrame=BaseFrame  EquilibriumPosition=0  EquilibriumPositionUnits=rad  SpringStiffness=0  SpringStiffnessUnits=N*m/rad  DampingCoefficient=0  DampingCoefficientUnits=N*m/(rad/s)  TorqueActuationMode=InputTorque  MotionActuationMode=ComputedMotion  SensePosition=off  SenseVelocity=on  SenseAcceleration=off  SenseTorqueForce=off  SenseLowerLimitTorqueForce=off  SenseUpperLimitTorqueForce=off  LowerLimitSpecify=off  LowerLimitBound=-90  LowerLimitBoundUnits=deg  LowerLimitStiffness=1e4  LowerLimitStiffnessUnits=N*m/deg  LowerLimitDamping=10  LowerLimitDampingUnits=N*m/(deg/s)  LowerLimitTransitionRegionWidth=0.1  LowerLimitTransitionRegionWidthUnits=deg  UpperLimitSpecify=off  UpperLimitBound=90  UpperLimitBoundUnits=deg  UpperLimitStiffness=1e4  UpperLimitStiffnessUnits=N*m/deg  UpperLimitDamping=10  UpperLimitDampingUnits=N*m/(deg/s)  UpperLimitTransitionRegionWidth=0.1  UpperLimitTransitionRegionWidthUnits=deg  PositionTargetSpecify=off  PositionTargetPriority=High  PositionTargetValue=0  PositionTargetValueUnits=deg  VelocityTargetSpecify=on  VelocityTargetPriority=High  VelocityTargetValue=initveh.Wheel.wFR  VelocityTargetValueUnits=rad/s
  Revolute RL : sm_lib/Joints/Revolute Joint  JointMode=Normal  SenseConstraintForce=off  SenseConstraintForceX=off  SenseConstraintForceY=off  SenseConstraintForceZ=off  SenseConstraintTorque=off  SenseConstraintTorqueX=off  SenseConstraintTorqueY=off  SenseConstraintTorqueZ=off  SenseTotalForce=off  SenseTotalForceX=off  SenseTotalForceY=off  SenseTotalForceZ=off  SenseTotalTorque=off  SenseTotalTorqueX=off  SenseTotalTorqueY=off  SenseTotalTorqueZ=off  CompositeWrenchDir=FollowerOnBase  CompositeWrenchFrame=BaseFrame  EquilibriumPosition=0  EquilibriumPositionUnits=rad  SpringStiffness=0  SpringStiffnessUnits=N*m/rad  DampingCoefficient=0  DampingCoefficientUnits=N*m/(rad/s)  TorqueActuationMode=InputTorque  MotionActuationMode=ComputedMotion  SensePosition=off  SenseVelocity=on  SenseAcceleration=off  SenseTorqueForce=off  SenseLowerLimitTorqueForce=off  SenseUpperLimitTorqueForce=off  LowerLimitSpecify=off  LowerLimitBound=-90  LowerLimitBoundUnits=deg  LowerLimitStiffness=1e4  LowerLimitStiffnessUnits=N*m/deg  LowerLimitDamping=10  LowerLimitDampingUnits=N*m/(deg/s)  LowerLimitTransitionRegionWidth=0.1  LowerLimitTransitionRegionWidthUnits=deg  UpperLimitSpecify=off  UpperLimitBound=90  UpperLimitBoundUnits=deg  UpperLimitStiffness=1e4  UpperLimitStiffnessUnits=N*m/deg  UpperLimitDamping=10  UpperLimitDampingUnits=N*m/(deg/s)  UpperLimitTransitionRegionWidth=0.1  UpperLimitTransitionRegionWidthUnits=deg  PositionTargetSpecify=off  PositionTargetPriority=High  PositionTargetValue=0  PositionTargetValueUnits=deg  VelocityTargetSpecify=on  VelocityTargetPriority=High  VelocityTargetValue=initveh.Wheel.wRL  VelocityTargetValueUnits=rad/s
  Revolute RR : sm_lib/Joints/Revolute Joint  JointMode=Normal  SenseConstraintForce=off  SenseConstraintForceX=off  SenseConstraintForceY=off  SenseConstraintForceZ=off  SenseConstraintTorque=off  SenseConstraintTorqueX=off  SenseConstraintTorqueY=off  SenseConstraintTorqueZ=off  SenseTotalForce=off  SenseTotalForceX=off  SenseTotalForceY=off  SenseTotalForceZ=off  SenseTotalTorque=off  SenseTotalTorqueX=off  SenseTotalTorqueY=off  SenseTotalTorqueZ=off  CompositeWrenchDir=FollowerOnBase  CompositeWrenchFrame=BaseFrame  EquilibriumPosition=0  EquilibriumPositionUnits=rad  SpringStiffness=0  SpringStiffnessUnits=N*m/rad  DampingCoefficient=0  DampingCoefficientUnits=N*m/(rad/s)  TorqueActuationMode=InputTorque  MotionActuationMode=ComputedMotion  SensePosition=off  SenseVelocity=on  SenseAcceleration=off  SenseTorqueForce=off  SenseLowerLimitTorqueForce=off  SenseUpperLimitTorqueForce=off  LowerLimitSpecify=off  LowerLimitBound=-90  LowerLimitBoundUnits=deg  LowerLimitStiffness=1e4  LowerLimitStiffnessUnits=N*m/deg  LowerLimitDamping=10  LowerLimitDampingUnits=N*m/(deg/s)  LowerLimitTransitionRegionWidth=0.1  LowerLimitTransitionRegionWidthUnits=deg  UpperLimitSpecify=off  UpperLimitBound=90  UpperLimitBoundUnits=deg  UpperLimitStiffness=1e4  UpperLimitStiffnessUnits=N*m/deg  UpperLimitDamping=10  UpperLimitDampingUnits=N*m/(deg/s)  UpperLimitTransitionRegionWidth=0.1  UpperLimitTransitionRegionWidthUnits=deg  PositionTargetSpecify=off  PositionTargetPriority=High  PositionTargetValue=0  PositionTargetValueUnits=deg  VelocityTargetSpecify=on  VelocityTargetPriority=High  VelocityTargetValue=initveh.Wheel.wRR  VelocityTargetValueUnits=rad/s
  Road Surface FL : sm_vehicle_utilities_lib/Road Surface  VariantControl=Choice  LabelModeActiveChoice=Flat  popup_leftRight=Left
      settings: AttributesFormatString=%<LabelModeActiveChoice>
  Road Surface FR : sm_vehicle_utilities_lib/Road Surface  VariantControl=Choice  LabelModeActiveChoice=Flat  popup_leftRight=Right
      settings: AttributesFormatString=%<LabelModeActiveChoice>
  Road Surface RL : sm_vehicle_utilities_lib/Road Surface  VariantControl=Choice  LabelModeActiveChoice=Flat  popup_leftRight=Left
      settings: AttributesFormatString=%<LabelModeActiveChoice>
  Road Surface RR : sm_vehicle_utilities_lib/Road Surface  VariantControl=Choice  LabelModeActiveChoice=Flat  popup_leftRight=Right
      settings: AttributesFormatString=%<LabelModeActiveChoice>
  Scene : Subsystem  Variant=on  VariantControlMode=label  LabelModeActiveChoice=Grid
      settings: AttributesFormatString=%<LabelModeActiveChoice>
      mask Display: disp(' ');
  Simulink-PS Converter{,1..3} (4 alike) : nesl_utility/Simulink-PS Converter  PhysicalDomain=network_engine_domain  SubClassName=ps_input  LeftPortType=input  RightPortType=output  PseudoPeriodic=off  Frequencies=[]  NoiseDistribution=none  NoiseParameters=[]  Unit=N*m  AffineConversion=off  FilteringAndDerivatives=provide  SimscapeFilterOrder=1  InputFilterTimeConstant=0.001  UdotUserProvided=0
  Suspension Front : Subsystem  mask(Suspension with Heave, Roll, and Ackerman Steering){zHeave=vehdata.SuspF.Heave.Height, kHeave=vehdata.SuspF.Heave.Stiffness, dHeave=vehdata.SuspF.Heave.Damping, xEqHeave=vehdata.SuspF.Heave.EqPos, zRoll=vehdata.SuspF.Roll.Height, kRoll=vehdata.SuspF.Roll.Stiffness, dRoll=vehdata.SuspF.Roll.Damping, aEqRoll=vehdata.SuspF.Roll.EqPos, mUnsprungMass=vehdata.SuspF.UnsprungMass.Mass, JUnsprungMass=vehdata.SuspF.UnsprungMass.Inertia, zUnsprungMass=vehdata.SuspF.UnsprungMass.Height, rUnsprungMass=vehdata.SuspF.UnsprungMass.Radius, lUnsprungMass=vehdata.SuspF.UnsprungMass.Length, zHub=vehdata.SuspF.Hub.Height, yTrack=vehdata.SuspF.Track, wheelbase=sum(abs(vehdata.Body.RA-vehdata.Body.FA)), steerRatio=vehdata.SuspF.SteerRatio}
      mask prompts: zHeave "Height (m)"; kHeave "Stiffness (N/m)"; dHeave "Damping (N/(m/s))"; xEqHeave "Equilibrium Position (m)"; zRoll "Height (m)"; kRoll "Stiffness (N*m/rad)"; dRoll "Damping (N*m/(rad/s)"; aEqRoll "Equilibrium Position (rad)"; mUnsprungMass "Mass (kg)"; JUnsprungMass "Inertia (kg*m^2)"; zUnsprungMass "Height (m)"; rUnsprungMass "Radius (m)"; lUnsprungMass "Length (m)"; zHub "Wheel Center Height (m)"; yTrack "Track Width (m)"; steerRatio "Steering Ratio"
      mask help: Models a suspension with heave and roll degrees of freedom for a single axle, with Ackermann steering. All heights are measured relative to the bottom of the wheels.
      settings: PortSchema="{\"entries\":[{\"content\":{\"sides\":[{\"content\":{\"connectorIds\":[\"LConn1\"]},\"type\":\"ConnectorPlacement.EquallySpacedRectSide\",\"uuid\":\"0af81f34-82de-4f02-a8a7-ec45be82faea\"},{\"content\":{\"connectorIds\":[\"In1\"],\"side\":\"RIGHT\"},\"type\":\"ConnectorPlacement.EquallySpacedRectSide\",\"uuid\":\"9bc48957-2707-4e2f-b988-a5743aaf8f58\"},{\"content\":{\"connectorIds\":[\"LConn2\"],\"side\":\"TOP\"},\"type\":\"ConnectorPlacement.EquallySpacedRectSide\",\"uuid\":\"08055243-2fee-46c8-8a4b-df5231c2978e\"},{\"content\":{\"connectorIds\":[\"RConn1\"],\"side\":\"BOTTOM\"},\"type\":\"ConnectorPlacement.EquallySpacedRectSide\",\"uuid\":\"745b1e5c-9113-4e99-a394-3eadcd3cd6f8\"}]},\"type\":\"ConnectorPlacement.EquallySpacedConnector\",\"uuid\":\"5011d399-f081-425d-a1fb-c00f3859766f\"}],\"packageUris\":[\"http://schema.mathworks.com/mf0/Connector/R2020b\"],\"version\":\"1.0\"}"
      mask DialogControl cont_heave_roll Prompt: Heave, Roll
      mask DialogControl group_heave Prompt: Heave
      mask DialogControl group_roll Prompt: Roll
      mask DialogControl cont_unsprung_mass Prompt: Unsprung Mass
      mask DialogControl cont_wheels_steering Prompt: Wheels, Steering
  Suspension Rear : Subsystem  mask(Suspension with Heave, Roll,){zHeave=vehdata.SuspR.Heave.Height, kHeave=vehdata.SuspR.Heave.Stiffness, dHeave=vehdata.SuspR.Heave.Damping, xEqHeave=vehdata.SuspR.Heave.EqPos, zRoll=vehdata.SuspR.Roll.Height, kRoll=vehdata.SuspR.Roll.Stiffness, dRoll=vehdata.SuspR.Roll.Damping, aEqRoll=vehdata.SuspR.Roll.EqPos, mUnsprungMass=vehdata.SuspR.UnsprungMass.Mass, JUnsprungMass=vehdata.SuspR.UnsprungMass.Inertia, zUnsprungMass=vehdata.SuspR.UnsprungMass.Height, rUnsprungMass=vehdata.SuspR.UnsprungMass.Radius, lUnsprungMass=vehdata.SuspR.UnsprungMass.Length, zHub=vehdata.SuspR.Hub.Height, yTrack=vehdata.SuspR.Track}
      mask prompts: zHeave "Height (m)"; kHeave "Stiffness (N/m)"; dHeave "Damping (N/(m/s))"; xEqHeave "Equilibrium Position (m)"; zRoll "Height (m)"; kRoll "Stiffness (N*m/rad)"; dRoll "Damping (N*m/(rad/s)"; aEqRoll "Equilibrium Position (rad)"; mUnsprungMass "Mass (kg)"; JUnsprungMass "Inertia (kg*m^2)"; zUnsprungMass "Height (m)"; rUnsprungMass "Radius (m)"; lUnsprungMass "Length (m)"; zHub "Wheel Center Height (m)"; yTrack "Track Width (m)"
      mask help: Models a suspension with heave and roll degrees of freedom for a single axle. All heights are measured relative to the bottom of the wheels.
      settings: PortSchema="{\"entries\":[{\"content\":{\"sides\":[{\"content\":{\"connectorIds\":[\"LConn1\"]},\"type\":\"ConnectorPlacement.EquallySpacedRectSide\",\"uuid\":\"0af81f34-82de-4f02-a8a7-ec45be82faea\"},{\"content\":{\"connectorIds\":[],\"side\":\"RIGHT\"},\"type\":\"ConnectorPlacement.EquallySpacedRectSide\",\"uuid\":\"9bc48957-2707-4e2f-b988-a5743aaf8f58\"},{\"content\":{\"connectorIds\":[\"LConn2\"],\"side\":\"TOP\"},\"type\":\"ConnectorPlacement.EquallySpacedRectSide\",\"uuid\":\"08055243-2fee-46c8-8a4b-df5231c2978e\"},{\"content\":{\"connectorIds\":[\"RConn1\"],\"side\":\"BOTTOM\"},\"type\":\"ConnectorPlacement.EquallySpacedRectSide\",\"uuid\":\"3fad50e5-0b96-4492-ad18-fd370deae0ca\"}]},\"type\":\"ConnectorPlacement.EquallySpacedConnector\",\"uuid\":\"5011d399-f081-425d-a1fb-c00f3859766f\"}],\"packageUris\":[\"http://schema.mathworks.com/mf0/Connector/R2020b\"],\"version\":\"1.0\"}"
      mask DialogControl cont_heave_roll Prompt: Heave, Roll
      mask DialogControl group_heave Prompt: Heave
      mask DialogControl group_roll Prompt: Roll
      mask DialogControl cont_unsprung_mass Prompt: Unsprung Mass
      mask DialogControl cont_wheels Prompt: Wheels
  Transform Scene : sm_lib/Frames and Transforms/Rigid Transform  TranslationMethod=None  TranslationStandardOffset=0  TranslationStandardOffsetUnits=m  TranslationStandardAxis=+Z  TranslationCartesianOffset=[0 0 0]  TranslationCartesianOffsetUnits=m  TranslationROffset=0  TranslationROffsetUnits=m  TranslationZOffset=0  TranslationZOffsetUnits=m  TranslationThetaOffset=0  TranslationThetaOffsetUnits=deg  RotationMethod=RotationSequence  RotationAngleUnits=deg  RotationStandardAxis=+Y  RotationAngle=0  RotationArbitraryAxis=[0 0 1]  FollAlignAxisA=+X  BaseAlignAxisA=+Y  FollAlignAxisB=+Y  BaseAlignAxisB=+Z  RotationSequenceAxes=FollowerAxes  RotationSequence=ZYX  RotationSequenceAngles=[SceneData.Reference.yaw SceneData.Reference.pitch SceneData.Reference.roll]  RotationSequenceAnglesUnits=rad  RotationMatrix=[1 0 0; 0 1 0; 0 0 1]  Quaternion=[1 0 0 0]
  Wheel FL : sm_vehicle_utilities_lib/Tire  popup_leftright=Left  tire_param=vehdata.TireDataF.param  rim_mass=vehdata.RimF.Mass  rim_inertia=vehdata.RimF.Inertia
  Wheel FR : sm_vehicle_utilities_lib/Tire  popup_leftright=Right  tire_param=vehdata.TireDataF.param  rim_mass=vehdata.RimF.Mass  rim_inertia=vehdata.RimF.Inertia
  Wheel RL : sm_vehicle_utilities_lib/Tire  popup_leftright=Left  tire_param=vehdata.TireDataR.param  rim_mass=vehdata.RimR.Mass  rim_inertia=vehdata.RimR.Inertia
  Wheel RR : sm_vehicle_utilities_lib/Tire  popup_leftright=Right  tire_param=vehdata.TireDataR.param  rim_mass=vehdata.RimR.Mass  rim_inertia=vehdata.RimR.Inertia
  World : Subsystem
  Out Bus Element9 : Outport  PortName=m  Element=Body
  Out Bus Element : Outport  PortName=m  Element=TireFL
  Out Bus Element1 : Outport  PortName=m  Element=TireFR
  Out Bus Element2 : Outport  PortName=m  Element=TireRL
  Out Bus Element3 : Outport  PortName=m  Element=TireRR
  Out Bus Element4 : Outport  PortName=m  Element=World
  wires:
  Wheel FL/1 -> [FL]
  Wheel RL/1 -> [RL]
  Wheel RR/1 -> [RR]
  Wheel FR/1 -> [FR]
  Bus Element In4/1 -> Suspension Front/1(s)
  Bus Element In/1 -> Simulink-PS Converter/1
  PS-Simulink Converter/1 -> [wFR]
  Bus Element In1/1 -> Simulink-PS Converter1/1
  PS-Simulink Converter1/1 -> [wRR]
  Bus Element In2/1 -> Simulink-PS Converter2/1
  PS-Simulink Converter2/1 -> [wRL]
  Bus Element In3/1 -> Simulink-PS Converter3/1
  PS-Simulink Converter3/1 -> [wFL]
  Body/1(m) -> Out Bus Element9/1
  [wFL] -> Outputs/1(wFL)
  [FL] -> Outputs/2(TFL)
  Outputs/1(FL) -> Out Bus Element/1
  [wFR] -> Outputs/3(wFR)
  [FR] -> Outputs/4(TFR)
  [wRL] -> Outputs/5(wRL)
  [RL] -> Outputs/6(TRL)
  [wRR] -> Outputs/7(wRR)
  [RR] -> Outputs/8(TRR)
  Outputs/2(FR) -> Out Bus Element1/1
  Outputs/3(RL) -> Out Bus Element2/1
  Outputs/4(RR) -> Out Bus Element3/1
  Body to World/1(World) -> Out Bus Element4/1
  Road Surface FL/1 -> Wheel FL/1
  Road Surface FR/1 -> Wheel FR/1
  Road Surface RR/1 -> Wheel RR/1
  Road Surface RL/1 -> Wheel RL/1
  connections:
  Body to World/LConn1 -- Transform Scene/LConn1 -- World/RConn1
  Body/LConn1 -- Suspension Rear/LConn1
  Wheel FR/LConn1 -- Road Surface FR/RConn1 -- Revolute FR/RConn1
  Suspension Front/RConn1 -- Revolute FR/LConn1
  Suspension Front/LConn2 -- Revolute FL/LConn1
  Suspension Rear/LConn2 -- Revolute RL/LConn1
  Revolute RR/LConn1 -- Suspension Rear/RConn1
  Wheel RL/LConn1 -- Road Surface RL/RConn1 -- Revolute RL/RConn1
  Camera Frames/RConn1 -- Body to World/RConn1 -- Body/RConn2
  Wheel FL/LConn1 -- Road Surface FL/RConn1 -- Revolute FL/RConn1
  Wheel RR/LConn1 -- Road Surface RR/RConn1 -- Revolute RR/RConn1
  Suspension Front/LConn1 -- Body/RConn1
  Revolute FR/RConn2 -- PS-Simulink Converter/LConn1
  Simulink-PS Converter/RConn1 -- Revolute FR/LConn2
  Simulink-PS Converter1/RConn1 -- Revolute RR/LConn2
  PS-Simulink Converter1/LConn1 -- Revolute RR/RConn2
  Simulink-PS Converter2/RConn1 -- Revolute RL/LConn2
  PS-Simulink Converter2/LConn1 -- Revolute RL/RConn2
  Simulink-PS Converter3/RConn1 -- Revolute FL/LConn2
  PS-Simulink Converter3/LConn1 -- Revolute FL/RConn2
  Scene/RConn1 -- Transform Scene/RConn1

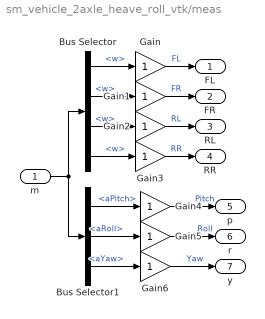
== system sm_vehicle_2axle_heave_roll_vtk/meas ==
  m : Inport
  Bus Selector : BusSelector  OutputSignals=TireFL.w,TireFR.w,TireRL.w,TireRR.w
  Bus Selector1 : BusSelector  OutputSignals=Body.aPitch,Body.aRoll,World.aYaw
  Gain{,1..6} (7 alike) : Gain
  FL : Outport
  FR : Outport  Port=2
  RL : Outport  Port=3
  RR : Outport  Port=4
  p : Outport  Port=5
  r : Outport  Port=6
  y : Outport  Port=7
  wires:
  Bus Selector/4 -> Gain3/1  "<w>"
  Bus Selector/2 -> Gain1/1  "<w>"
  Bus Selector/3 -> Gain2/1  "<w>"
  Bus Selector/1 -> Gain/1  "<w>"
  m/1 -> Bus Selector/1, Bus Selector1/1
  Gain3/1 -> RR/1  "RR"
  Gain/1 -> FL/1  "FL"
  Gain1/1 -> FR/1  "FR"
  Gain2/1 -> RL/1  "RL"
  Bus Selector1/1 -> Gain4/1  "<aPitch>"
  Bus Selector1/2 -> Gain5/1  "<aRoll>"
  Bus Selector1/3 -> Gain6/1  "<aYaw>"
  Gain6/1 -> y/1  "Yaw"
  Gain5/1 -> r/1  "Roll"
  Gain4/1 -> p/1  "Pitch"

== system sm_vehicle_2axle_heave_roll_vtk/Driver Input/External ==
  u : Inport
  Drv : Outport
  wires:
  u/1 -> Drv/1
